simulink model "w4"  (R2020b)
settings: Solver=VariableStepAuto  StartTime=0.0  StopTime=10.0  RelTol=1e-3
undefined symbols (not defined in the file or in its folder): gfprimfd
libraries: commblkcod2 x2, commrandsrc3 x1, commsink2 x1
settings Model: Creator=雨后星空  LastModifiedBy=雨后星空

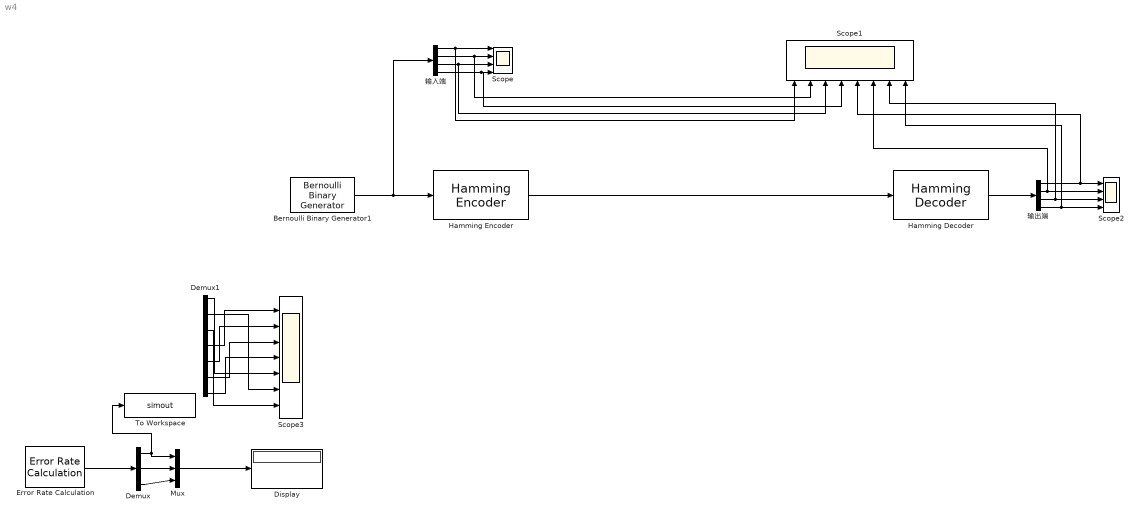
== system w4 ==
  Bernoulli Binary Generator1 : commrandsrc3/Bernoulli Binary Generator  ProbabilityOfZero=0.5  SeedSource=Parameter  Seed=67  SampleTime=0.05  SamplesPerFrame=4  OutputDataType=double  SimulateUsing=Interpreted execution
  Demux : Demux  Outputs=3
  Demux1 : Demux  Outputs=7
  Display : Display
  Error Rate Calculation : commsink2/Error Rate Calculation  N=0  st_delay=0  cp_mode=Entire frame  subframe=[]  PMode=Port  WsName=ErrorVec  RsMode2=off  stop=off  numErr=100  maxBits=1e6
      settings: SourceProductName=Communications Toolbox
  Hamming Decoder : commblkcod2/Hamming Decoder  n=7  k=gfprimfd(3,'min')
      settings: SourceProductBaseCode=CM
  Hamming Encoder : commblkcod2/Hamming Encoder  n=7  k=gfprimfd(3,'min')
      settings: SourceProductBaseCode=CM
  Mux : Mux  Inputs=3
  Scope : Scope  NumInputPorts=4
  Scope1 : Scope  NumInputPorts=8
  Scope2 : Scope  NumInputPorts=4
  Scope3 : Scope  NumInputPorts=7
  To Workspace : ToWorkspace  VariableName=simout  SampleTime=-1
  输入端 : Demux
  输出端 : Demux
  wires:
  Bernoulli Binary Generator1/1 -> 输入端/1, Hamming Encoder/1
  Hamming Encoder/1 -> Hamming Decoder/1
  Demux/1 -> Mux/1, To Workspace/1
  Demux1/2 -> Scope3/6
  Demux1/4 -> Scope3/1
  Demux1/1 -> Scope3/5
  Demux1/6 -> Scope3/3
  Demux1/3 -> Scope3/7
  Demux1/5 -> Scope3/2
  Demux1/7 -> Scope3/4
  Demux/2 -> Mux/2
  Demux/3 -> Mux/3
  Mux/1 -> Display/1
  Hamming Decoder/1 -> 输出端/1
  输出端/4 -> Scope2/4, Scope1/8
  输出端/3 -> Scope2/3, Scope1/7
  输出端/2 -> Scope2/2, Scope1/6
  输出端/1 -> Scope1/5, Scope2/1
  输入端/1 -> Scope1/1, Scope/1
  输入端/2 -> Scope1/2, Scope/2
  输入端/3 -> Scope1/3, Scope/3
  输入端/4 -> Scope1/4, Scope/4
  Error Rate Calculation/1 -> Demux/1
